simulink library "tqd"  (R2021b)
settings: Solver=VariableStepAuto  StartTime=0.0  StopTime=10.0  RelTol=1e-3
undefined symbols (not defined in the file or in its folder): ATQD_APSDecReq_X_kph, ATQD_APSDecReq_Y_mps2, ATQD_APSDecReqCMD_X_kph, ATQD_APSDecReqTs_X_pct, ATQD_APSDecTimeGain_X_Deg, ATQD_APSDecTimeGain_Y_s, ATQD_APSReqLowSpd_X_Deg, ATQD_AutoHoldReleaseBPS_X_Deg, ATQD_AWDLoadTrqnsGain_X_kg, ATQD_AWDLoadTrqnsGain_Y_pct, ATQD_BOSEnBPSPosn_X_kph, ATQD_BOSMap_X_rpm, ATQD_BOSMap_Y_pct, ATQD_CreepBaseTqD_X_kph, ATQD_CreepBaseTqD_Y_Deg, ATQD_CreepBaseTqR_X_kph, ATQD_CreepBaseTqR_Y_Deg, ATQD_CreepBPSDisPosn_X_Deg, ATQD_CreepBPSDisPosnR_X_Deg, ATQD_CreepBPSEnPosn_X_Deg, ATQD_CreepBPSEnPosnR_X_Deg, ATQD_CreepDeltaTq_X_kph, ATQD_CreepIterm_X_kph, ATQD_CreepIterm_Y_kph, ATQD_CreepItermMaxLimit_X_pct, ATQD_CreepPreloadTime_X_kph, ATQD_CreepPreloadTq_X_kph, ATQD_CreepPreloadTq_Y_s, ATQD_CreepProtTq_X_Deg, ATQD_CreepPterm_X_kph, ATQD_ECOTqMapD_X_rpm, ATQD_ECOTqMapD_Y_pct, ATQD_EOPDTqMapDCon_X_rpm, ATQD_EOPDTqMapDCon_Y_Deg, ATQD_EstInitVehWeight_X_c, ATQD_LHMRollGenMapD_X_rpm, ATQD_LHMRollGenMapD_Y_rpm, ATQD_LHMTqMapD_X_rpm, ATQD_LHMTqMapD_Y_pct, ATQD_NL1TqMapD_X_rpm, ATQD_NL1TqMapD_Y_pct, ATQD_NOPDTqMapDCon_X_rpm, ATQD_NOPDTqMapDCon_Y_Deg, ATQD_NRMRrEDUSpRat_X_rpm, ATQD_NRMRrEDUSpRat_Y_Nm, ATQD_OPDHoldDownRelDelay_X_Deg, ATQD_OPDHoldEnSpd_X_Deg, ATQD_OPDHoldRelDetTime_X_Deg, ATQD_OPDHoldReleaseTq_X_Deg, ATQD_OrigPedTqLowLim_X_Deg, ATQD_OrigPedTqLowLim_Y_pct, ATQD_PedalMapClimbUpLim_X_rpm, ATQD_PedalMapClimbUpLim_Y_Deg, ATQD_PreLoadTq_X_s, ATQD_RollGenMapEL1_X_rpm, ATQD_RollGenMapEL1_Y_rpm, ATQD_SL1TqMapD_X_rpm, ATQD_SL1TqMapD_Y_pct, ATQD_SlideRegenTqGain_X_Gps, ATQD_SlideRegenTqGain_Y_pct ... (+444)
libraries: hcu_lib x70, simulink x61, tqr x1
(part 1 of 14)
settings Model: Creator=13615  LastModifiedBy=FVT23010
settings SolverCC: AlgebraicLoopSolver=TrustRegion
settings DataIOCC: SaveFormat=Array  SignalLoggingSaveFormat=ModelDataLogs  ReturnWorkspaceOutputs=off
settings OptimizationCC: BlockReduction=off  BooleanDataType=off
settings DebuggingCC: SaveWithParameterizedLinksMsg=none  UnderspecifiedInitializationDetection=Classic  MergeDetectMultiDrivingBlocksExec=none  SignalResolutionControl=TryResolveAllWithWarning
settings HardwareCC: TargetUnknown=on
settings ModelReferenceCC: PropagateSignalLabelsOutOfModel=off
settings SFSimCC: SimUseLocalCustomCode=off
settings RTWCC: RTWUseLocalCustomCode=off
settings ConfigComp: CovMetricSettings=dw  CovSaveCumulativeToWorkspaceVar=on  CovSaveSingleToWorkspaceVar=on

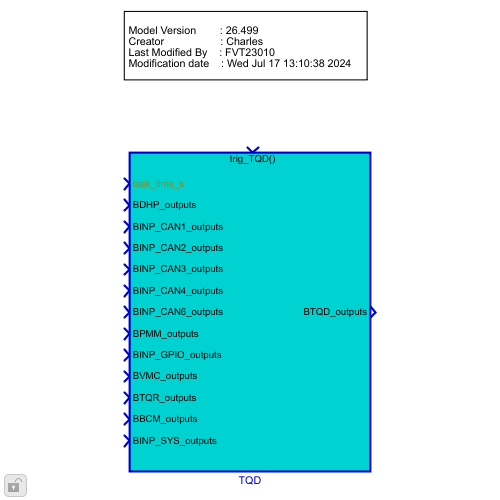
[thumbnail: Simulink's stored preview of the top-level diagram]
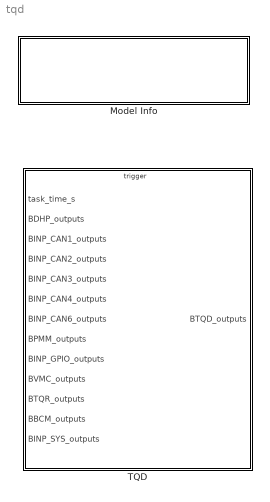
== system tqd ==
  Model Info : Subsystem  LoadFcn=slcm LoadBlock;  InitFcn=slcm('UpdateAllCMBlocksInThisModelInit')  mask(CMBlock){InitialSaveTempField=, InitialBlockCM=None, BlockCM=None, Frame=on, SaveTempField=, DisplayStringWithTags=|, MaskDisplayString=Model Version        : 26.504\nCreator                   : Charles\nLast Modified By    : FVT23010\nModification date    : Thu Jul 18 10:59:55 2024, HorizontalTextAlignment=Left, LeftAlignmentValue=0.02, SourceBlockDiagram=tqd, TagMaxNumber=20, CMTag1=, CMTag2=, CMTag3=, CMTag4=, CMTag5=, CMTag6=, CMTag7=, CMTag8=, CMTag9=, CMTag10=, CMTag11=, CMTag12=, CMTag13=, CMTag14=, CMTag15=, CMTag16=, CMTag17=, CMTag18=, CMTag19=, CMTag20=}
      mask DisplayStringWithTags=|
      | Model Version        : %<ModelVersion>
      | Creator                   : Charles
      | Last Modified By    : %<LastModifiedBy>
      | Modification date    : %<LastModificationDate>
      mask help: This block allows revision control information to be displayed within the model.
      settings: CopyFcn=slcm CopyBlock;  DeleteFcn=slcm Cancel;  PostSaveFcn=slcm('UpdateAllCMBlocksInThisModel')  NameChangeFcn=slcm Rename;  OpenFcn=slcm
      mask Display: text(str2num(LeftAlignmentValue), 0.5, MaskDisplayString, 'HorizontalAlignment', HorizontalTextAlignment)
  TQD : Subsystem
      settings: RTWSystemCode=Nonreusable function  RTWFcnNameOpts=Use subsystem name  RTWFileNameOpts=Use subsystem name

== system tqd/Model Info ==
  EmptySubsystem : Subsystem

== system tqd/TQD ==
  task_time_s : Inport
  BDHP_outputs : Inport  Port=2  OutDataTypeStr=Bus: BDHP_outputs
  BINP_CAN1_outputs : Inport  Port=3  OutDataTypeStr=Bus: BINP_CAN1_outputs
  BINP_CAN2_outputs : Inport  Port=4  OutDataTypeStr=Bus: BINP_CAN2_outputs
  BINP_CAN3_outputs : Inport  Port=5  OutDataTypeStr=Bus: BINP_CAN3_outputs
  BINP_CAN4_outputs : Inport  Port=6  OutDataTypeStr=Bus: BINP_CAN4_outputs
  BINP_CAN6_outputs : Inport  Port=7  OutDataTypeStr=Bus: BINP_CAN6_outputs
  BPMM_outputs : Inport  Port=8  OutDataTypeStr=Bus: BPMM_outputs
  BINP_GPIO_outputs : Inport  Port=9  OutDataTypeStr=Bus: BINP_GPIO_outputs
  BVMC_outputs : Inport  Port=10  OutDataTypeStr=Bus: BVMC_outputs
  BTQR_outputs : Inport  Port=11  OutDataTypeStr=Bus: BTQR_outputs  LockScale=on
  BBCM_outputs : Inport  Port=12  OutDataTypeStr=Bus: BBCM_outputs
  BINP_SYS_outputs : Inport  Port=13  OutDataTypeStr=Bus: BINP_SYS_outputs
  trig_TQD : TriggerPort  TriggerType=function-call  VariantControl=(inherit)
  Bus Creator2 : BusCreator  Inputs=87  OutDataTypeStr=Bus: BTQD_outputs  NonVirtualBus=on
  Bus Selector : BusSelector  OutputSignals=VINP_IVIPWModeReq_enum,VINP_IVICreepSWReq_flg,VINP_RollModeSWCmd_enum,VINP_IVIPwrLockSW_enum,VINP_IVIISAOffsetSpd_enum,VINP_Distanceunit_flg
  Bus Selector1 : BusSelector  OutputSignals=VDHP_ActAPSPosn_pct,VDHP_LowIdleAccPedal_flg
  Bus Selector10 : BusSelector  OutputSignals=VBCM_BrakeLamp_flg
  Bus Selector11 : BusSelector  OutputSignals=VINP_FlashRegenMode_enum
  Bus Selector12 : BusSelector  OutputSignals=VINP_ShifterHandleCmd_enum,VINP_FrEDURotateDirction_enum,VINP_RrEDURotateDirction_enum,VINP_FrTMSpd_rpm,VINP_RrTMSpd_rpm,VINP_HVBPwrAvailDchrg_kW,VINP_HVBPwrAvailChrg_kW,VINP_FrRegenAvailTq_Nm,VINP_RrRegenAvailTq_Nm,VINP_FrEDURealTMTq_Nm,VINP_RrEDURealTMTq_Nm,VINP_HVBattErr_flg,VINP_DCDCFaultSta_enum,VINP_FrMotorAvailTq_Nm,VINP_RrMotorAvailTq_Nm,VINP_MCUWarnF_enum,VINP_MCUWarnR_enum,VINP_ChrgPlugSta_enum,VINP_HVBCellVoltMax_mV,VINP_HVBCellVoltMin_mV,VINP_HVBSOH_pct,VINP_HVBattSOC_pct
  Bus Selector2 : BusSelector  OutputSignals=VINP_VehSpeed_kph,VINP_BrkSwSta_flg,VINP_BrkSwV_flg,VINP_BrkPedalPos_pct,VINP_BrkPedalPosSta_flg,VINP_FrPTCSActive_flg,VINP_RrPTCSActive_flg,VINP_FrntAxlTrqReqDrv_Nm,VINP_RearAxlTrqReqDrv_Nm,VINP_FrRBCActive_flg,VINP_RrRBCActive_flg,VINP_FrntAxlTrqReqBrk_Nm,VINP_RearAxlTrqReqBrk_Nm,VINP_CrashOutputSts_enum,VINP_LongAccel_Gps,VINP_EPBCarWashMode_flg,VINP_EPBErrSta_enum,VINP_EPBSta_enum,VINP_DOASta_flg,VINP_GRADE_Deg,VINP_HSAActive_flg,VINP_DriverSeatBeltCmd_flg,VINP_AVHActive_flg,VINP_PsngrSeatBeltCmd_flg,VINP_RDriverSeatBeltCmd_flg,VINP_RCenterSeatBeltCmd_flg,VINP_RPsngrSeatBeltCmd_flg,VINP_YawRate_degps,VINP_SASAngle_Deg,VINP_MCPressure_bar
  Bus Selector3 : BusSelector  OutputSignals=VINP_BrakeSWGPIO_flg,VINP_CrashSignalGPIO_flg,VINP_DrDoorSW_flg,VINP_SeatSW_flg,VINP_HoodSW_flg,VINP_TailgateSW_flg,VINP_PsDoorSW_flg,VINP_RRDoorSW_flg,VINP_RLDoorSW_flg
  Bus Selector5 : BusSelector  OutputSignals=VVMC_ADASForceIdle_flg,VVMC_ACCRequiredAccel_mps2,VVMC_ACCVehHoldReq_flg,VVMC_ADASActive_flg,VVMC_ADASWhlTqReq_Nm,VVMC_CruzActive_flg,VVMC_CruzWhlTqReq_Nm,VVMC_MSAActive_flg,VVMC_MSAWhlTqReq_Nm,VVMC_APSActive_flg,VVMC_APSSpeedCMD_kph,VVMC_APSShiftPosnReq_enum,VVMC_ACCPedalOvrd_flg,VVMC_LongAcc_Gps,VVMC_ActMaxSlideRate_pct,VVMC_EstSlope_Deg,VVMC_APSReq_enum,VVMC_RWDRDCActive_enum,VVMC_ActLRSlideRate_pct,VVMC_ActRRSlideRate_pct,VVMC_ActStESCYaw_Dps,VVMC_CCCtrlSta_enum,VVMC_MSACtrlSta_enum,VVMC_LVDAACCStatusInformation_flg,VVMC_ACCObjDist_m,VVMC_MeterIndSpeed_raw32,VVMC_RearTqRatio_rat,VVMC_ACCOvrdMemTq_Nm,VVMC_CalibratedGyroY_Dps,VVMC_CAASActive_flg
  Bus Selector6 : BusSelector  OutputSignals=VINP_SWCResUpSta_flg,VINP_SWCSetdownSta_flg,VINP_SWCACCSta_flg,VINP_SWCCANCELSta_flg,VINP_SWCRegenUp_flg,VINP_SWCRegenDown_flg
  Bus Selector7 : BusSelector  OutputSignals=VPMM_PowerSta_enum,VPMM_DrivetrainSelect_enum,VPMM_SysPowerMode_enum
  Bus Selector8 : BusSelector  OutputSignals=VTQR_ActualFEDUWhlTqReq_Nm,VTQR_ActualREDUWhlTqReq_Nm,VTQR_NoABSFEDUWhlTqReq_Nm,VTQR_NoABSREDUWhlTqReq_Nm
  Bus Selector9 : BusSelector  OutputSignals=VINP_ADASISASta_enum,VINP_ADASVehSpdLim_enum,VINP_ADASACCSta_enum
  Data Type Conversion : DataTypeConversion  OutDataTypeStr=uint8
  Data Type Conversion1 : DataTypeConversion  OutDataTypeStr=uint8
  Data Type Conversion2 : DataTypeConversion  OutDataTypeStr=boolean
  Data Type Conversion3 : DataTypeConversion  OutDataTypeStr=boolean
  Ground{,1..3} (4 alike) : Ground
  TorqueDemand : Subsystem
  BTQD_outputs : Outport  OutDataTypeStr=Bus: BTQD_outputs
  wires:
  Bus Selector2/19 -> TorqueDemand/25(VINP_DOASta_flg)  "<VINP_DOASta_flg>"
  Bus Selector2/18 -> TorqueDemand/24(VINP_EPBSta_enum)  "<VINP_EPBSta_enum>"
  Bus Selector2/17 -> TorqueDemand/23(VINP_EPBErrSta_enum)  "<VINP_EPBErrSta_enum>"
  Bus Selector2/16 -> TorqueDemand/22(VINP_EPBCarWashMode_flg)  "<VINP_EPBCarWashMode_flg>"
  Bus Selector2/15 -> TorqueDemand/21(VINP_LongAccel_Gps)  "<VINP_LongAccel_Gps>"
  BTQR_outputs/1 -> Bus Selector8/1
  Bus Selector2/14 -> TorqueDemand/20(VINP_CrashOutputSts_enum)  "<VINP_CrashOutputSts_enum>"
  TorqueDemand/8(VTQD_TqSourceFr_enum) -> Bus Creator2/8
  BDHP_outputs/1 -> Bus Selector1/1
  Bus Selector2/5 -> TorqueDemand/11(VINP_BrkPedalPosSta_flg)  "<VINP_BrkPedalPosSta_flg>"
  TorqueDemand/10(VTQD_FrEDUAvailBrkRgnTq_Nm) -> Bus Creator2/10
  TorqueDemand/9(VTQD_TqSourceRr_enum) -> Bus Creator2/9
  TorqueDemand/7(VTQD_AfterAvailableTqDemRr_Nm) -> Bus Creator2/7
  TorqueDemand/6(VTQD_AfterAvailableTqDemFr_Nm) -> Bus Creator2/6
  TorqueDemand/5(VTQD_DriverWhlTqDem_Nm) -> Bus Creator2/5
  Bus Selector/1 -> TorqueDemand/37(VINP_IVIPWModeReq_enum)  "<VINP_IVIPWModeReq_enum>"
  TorqueDemand/4(VTQD_PBWUnlockTO_flg) -> Bus Creator2/4
  TorqueDemand/3(VTQD_PBWLockTO_flg) -> Bus Creator2/3
  TorqueDemand/2(VTQD_ParkRequest_flg) -> Bus Creator2/2
  TorqueDemand/1(VTQD_GearActualPosn_enum) -> Bus Creator2/1
  BINP_CAN4_outputs/1 -> Bus Selector6/1  "BINP_CAN4_outputs"
  BINP_CAN2_outputs/1 -> Bus Selector/1  "BINP_CAN2_outputs"
  Bus Selector2/11 -> TorqueDemand/17(VINP_RrRBCActive_flg)  "<VINP_RrRBCActive_flg>"
  Bus Selector2/7 -> TorqueDemand/13(VINP_RrPTCSActive_flg)  "<VINP_RrPTCSActive_flg>"
  Bus Selector7/2 -> TorqueDemand/5(VPMM_DrivetrainSelect_enum)  "<VPMM_DrivetrainSelect_enum>"
  BINP_GPIO_outputs/1 -> Bus Selector3/1
  Bus Selector1/2 -> TorqueDemand/3(VDHP_LowIdleAccPedal_flg)  "<VDHP_LowIdleAccPedal_flg>"
  Bus Selector1/1 -> TorqueDemand/2(VDHP_ActAPSPosn_pct)  "<VDHP_ActAPSPosn_pct>"
  Bus Selector2/10 -> TorqueDemand/16(VINP_FrRBCActive_flg)  "<VINP_FrRBCActive_flg>"
  Bus Selector2/9 -> TorqueDemand/15(VINP_RearAxlTrqReqDrv_Nm)  "<VINP_RearAxlTrqReqDrv_Nm>"
  Bus Selector2/8 -> TorqueDemand/14(VINP_FrntAxlTrqReqDrv_Nm)  "<VINP_FrntAxlTrqReqDrv_Nm>"
  Bus Selector2/13 -> TorqueDemand/19(VINP_RearAxlTrqReqBrk_Nm)  "<VINP_RearAxlTrqReqBrk_Nm>"
  Bus Selector2/12 -> TorqueDemand/18(VINP_FrntAxlTrqReqBrk_Nm)  "<VINP_FrntAxlTrqReqBrk_Nm>"
  Bus Selector2/4 -> TorqueDemand/10(VINP_BrkPedalPos_pct)  "<VINP_BrkPedalPos_pct>"
  Bus Selector2/3 -> TorqueDemand/9(VINP_BrkSwV_flg)  "<VINP_BrkSwV_flg>"
  Bus Selector2/2 -> TorqueDemand/8(VINP_BrkSwSta_flg)  "<VINP_BrkSwSta_flg>"
  Bus Selector2/1 -> TorqueDemand/7(VINP_VehSpeed_kph)  "<VINP_VehSpeed_kph>"
  Bus Selector2/6 -> TorqueDemand/12(VINP_FrPTCSActive_flg)  "<VINP_FrPTCSActive_flg>"
  Bus Selector7/1 -> TorqueDemand/4(VPMM_PowerSta_enum)  "<VPMM_PowerSta_enum>"
  task_time_s/1 -> TorqueDemand/1(task_time_s)  "task_time_s"
  BINP_CAN3_outputs/1 -> Bus Selector12/1
  BINP_CAN1_outputs/1 -> Bus Selector2/1
  BPMM_outputs/1 -> Bus Selector7/1
  Bus Creator2/1 -> BTQD_outputs/1  "BTQD_outputs"
  Bus Selector2/20 -> TorqueDemand/26(VINP_GRADE_Deg)  "<VINP_GRADE_Deg>"
  Bus Selector2/21 -> TorqueDemand/27(VINP_HSAActive_flg)  "<VINP_HSAActive_flg>"
  Bus Selector/2 -> TorqueDemand/38(VINP_IVICreepSWReq_flg)  "<VINP_IVICreepSWReq_flg>"
  Bus Selector2/22 -> TorqueDemand/28(VINP_DriverSeatBeltCmd_flg)  "<VINP_DriverSeatBeltCmd_flg>"
  Bus Selector7/3 -> TorqueDemand/6(VPMM_SysPowerMode_enum)  "<VPMM_SysPowerMode_enum>"
  Bus Selector2/23 -> TorqueDemand/29(VINP_AVHActive_flg)  "<VINP_AVHActive_flg>"
  Bus Selector2/24 -> TorqueDemand/30(VINP_PsngrSeatBeltCmd_flg)  "<VINP_PsngrSeatBeltCmd_flg>"
  Bus Selector2/25 -> TorqueDemand/31(VINP_RDriverSeatBeltCmd_flg)  "<VINP_RDriverSeatBeltCmd_flg>"
  Bus Selector2/27 -> TorqueDemand/33(VINP_RPsngrSeatBeltCmd_flg)  "<VINP_RPsngrSeatBeltCmd_flg>"
  Bus Selector/3 -> TorqueDemand/39(VINP_RollModeSWCmd_enum)  "<VINP_RollModeSWCmd_enum>"
  Bus Selector2/26 -> TorqueDemand/32(VINP_RCenterSeatBeltCmd_flg)  "<VINP_RCenterSeatBeltCmd_flg>"
  Bus Selector6/1 -> TorqueDemand/65(VINP_SWCResUpSta_flg)  "<VINP_SWCResUpSta_flg>"
  Bus Selector/4 -> TorqueDemand/40(VINP_IVIPwrLockSW_enum)  "<VINP_IVIPwrLockSW_enum>"
  Ground2/1 -> Data Type Conversion/1
  Bus Selector2/28 -> TorqueDemand/34(VINP_YawRate_degps)  "<VINP_YawRate_degps>"
  Bus Selector2/29 -> TorqueDemand/35(VINP_SASAngle_Deg)  "<VINP_SASAngle_Deg>"
  Bus Selector2/30 -> TorqueDemand/36(VINP_MCPressure_bar)  "<VINP_MCPressure_bar>"
  TorqueDemand/11(VTQD_RrEDUAvailBrkRgnTq_Nm) -> Bus Creator2/11
  TorqueDemand/12(VTQD_TqTargetShaftSpd_rpm) -> Bus Creator2/12
  TorqueDemand/13(VTQD_LimpHomeAct_flg) -> Bus Creator2/13
  TorqueDemand/14(VTQD_RollRegenEnable_flg) -> Bus Creator2/14
  TorqueDemand/15(VTQD_EVDriveMode_enum) -> Bus Creator2/15
  TorqueDemand/16(VTQD_EVDriveModeValid_flg) -> Bus Creator2/16
  TorqueDemand/17(VTQD_ShiftGearPosn_enum) -> Bus Creator2/17
  TorqueDemand/18(VTQD_PButtonSta_enum) -> Bus Creator2/18
  TorqueDemand/19(VTQD_FrActvDmpDisabReq_flg) -> Bus Creator2/19
  TorqueDemand/20(VTQD_RrActvDmpDisabReq_flg) -> Bus Creator2/20
  TorqueDemand/21(VTQD_FrRgnDecrSta_flg) -> Bus Creator2/21
  TorqueDemand/22(VTQD_RrRgnDecrSta_flg) -> Bus Creator2/22
  TorqueDemand/23(VTQD_DriverWhlTqDemFr_Nm) -> Bus Creator2/23
  TorqueDemand/24(VTQD_DriverWhlTqDemRr_Nm) -> Bus Creator2/24
  TorqueDemand/25(VTQD_FrEDUActTq_Nm) -> Bus Creator2/25
  TorqueDemand/26(VTQD_RrEDUActTq_Nm) -> Bus Creator2/26
  TorqueDemand/27(VTQD_FrEDURolRgnTq_Nm) -> Bus Creator2/27
  TorqueDemand/28(VTQD_RrEDURolRgnTq_Nm) -> Bus Creator2/28
  TorqueDemand/29(VTQD_FrEDUSpd_rpm) -> Bus Creator2/29
  TorqueDemand/30(VTQD_RrEDUSpd_rpm) -> Bus Creator2/30
  TorqueDemand/31(VTQD_FrEDUSpdValid_flg) -> Bus Creator2/31
  TorqueDemand/32(VTQD_FrEDUAvailBrkRgnTqV_flg) -> Bus Creator2/32
  TorqueDemand/33(VTQD_RrEDUSpdValid_flg) -> Bus Creator2/33
  TorqueDemand/34(VTQD_RrEDUAvailBrkRgnTqV_flg) -> Bus Creator2/34
  TorqueDemand/35(VTQD_RgnAbnorSta_flg) -> Bus Creator2/35
  TorqueDemand/36(VTQD_PTCSPermSta_flg) -> Bus Creator2/36
  TorqueDemand/37(VTQD_FrRgnPermSta_flg) -> Bus Creator2/37
  TorqueDemand/38(VTQD_RrRgnPermSta_flg) -> Bus Creator2/38
  TorqueDemand/39(VTQD_ExternalTqAllow_flg) -> Bus Creator2/39
  TorqueDemand/40(VTQD_FrIdcMin_A) -> Bus Creator2/40
  TorqueDemand/41(VTQD_FrIdcMax_A) -> Bus Creator2/41
  TorqueDemand/42(VTQD_FrUdcMin_V) -> Bus Creator2/42
  TorqueDemand/43(VTQD_FrUdcMax_V) -> Bus Creator2/43
  TorqueDemand/44(VTQD_RrIdcMin_A) -> Bus Creator2/44
  TorqueDemand/45(VTQD_RrIdcMax_A) -> Bus Creator2/45
  TorqueDemand/46(VTQD_RrUdcMin_V) -> Bus Creator2/46
  TorqueDemand/47(VTQD_RrUdcMax_V) -> Bus Creator2/47
  TorqueDemand/48(VTQD_CoordWhlTqDemFr_Nm) -> Bus Creator2/48
  TorqueDemand/49(VTQD_CoordWhlTqDemRr_Nm) -> Bus Creator2/49
  TorqueDemand/50(VTQD_CreepEnable_flg) -> Bus Creator2/50
  TorqueDemand/51(VTQD_CrashDetd_flg) -> Bus Creator2/51
  TorqueDemand/52(VTQD_DiagHCrash_flg) -> Bus Creator2/52
  TorqueDemand/53(VTQD_ReBrakeLPReq_flg) -> Bus Creator2/53
  TorqueDemand/54(VTQD_LoSpdBrkCtrl_flg) -> Bus Creator2/54
  TorqueDemand/55(VTQD_LowIdleAccPedal_flg) -> Bus Creator2/55
  TorqueDemand/56(VTQD_APSStaSys_enum) -> Bus Creator2/56
  TorqueDemand/57(VTQD_APSReq_enum) -> Bus Creator2/57
  TorqueDemand/58(VTQD_APSDecReqA_flg) -> Bus Creator2/58
  TorqueDemand/59(VTQD_APSDecReq_mps2) -> Bus Creator2/59
  TorqueDemand/60(VTQD_ExtShftAllow_flg) -> Bus Creator2/60
  TorqueDemand/61(VTQD_EstVehWeightResult_kg) -> Bus Creator2/61
  TorqueDemand/62(VTQD_BOSEnable_flg) -> Bus Creator2/62
  TorqueDemand/63(VTQD_CreepON_flg) -> Bus Creator2/63
  TorqueDemand/64(VTQD_PreLoadHold_flg) -> Bus Creator2/64
  TorqueDemand/65(VTQD_PreLoadPreEn_flg) -> Bus Creator2/65
  TorqueDemand/66(VTQD_CreepPrLoadEnable_flg) -> Bus Creator2/66
  TorqueDemand/67(VTQD_RDCActive_enum) -> Bus Creator2/67
  TorqueDemand/68(VTQD_EquivAccPedalSWSta_flg) -> Bus Creator2/68
  TorqueDemand/69(VTQD_DriveProtEn_flg) -> Bus Creator2/69
  TorqueDemand/70(VTQD_ActParkRequest_flg) -> Bus Creator2/70
  TorqueDemand/71(VTQD_RegenTqLimitEn_flg) -> Bus Creator2/71
  TorqueDemand/72(VTQD_PedAccTqEn_flg) -> Bus Creator2/72
  TorqueDemand/73(VTQD_IVIPwrLockSta_enum) -> Bus Creator2/73
  TorqueDemand/74(VTQD_ExtDoorAllow_flg) -> Bus Creator2/74
  TorqueDemand/75(VTQD_WhlTqCapGenFr_Nm) -> Bus Creator2/75
  TorqueDemand/76(VTQD_WhlTqCapGenRr_Nm) -> Bus Creator2/76
  TorqueDemand/77(VTQD_OPDHoldLamp_flg) -> Bus Creator2/77
  TorqueDemand/78(VTQD_RegenMode_enum) -> Bus Creator2/78
  BINP_CAN6_outputs/1 -> Bus Selector9/1
  Bus Selector/5 -> TorqueDemand/41(VINP_IVIISAOffsetSpd_enum)  "<VINP_IVIISAOffsetSpd_enum>"
  BBCM_outputs/1 -> Bus Selector10/1
  Bus Selector6/2 -> TorqueDemand/66(VINP_SWCSetdownSta_flg)  "<VINP_SWCSetdownSta_flg>"
  Bus Selector6/3 -> TorqueDemand/67(VINP_SWCACCSta_flg)  "<VINP_SWCACCSta_flg>"
  Bus Selector6/4 -> TorqueDemand/68(VINP_SWCCANCELSta_flg)  "<VINP_SWCCANCELSta_flg>"
  Bus Selector6/5 -> TorqueDemand/69(VINP_SWCRegenUp_flg)  "<VINP_SWCRegenUp_flg>"
  Bus Selector6/6 -> TorqueDemand/70(VINP_SWCRegenDown_flg)  "<VINP_SWCRegenDown_flg>"
  TorqueDemand/79(VTQD_SaveRegenMode_enum) -> Bus Creator2/79
  TorqueDemand/80(VTQD_FDCVCURegenMode_enum) -> Bus Creator2/80
  TorqueDemand/81(VTQD_SpdCtrlMode_enum) -> Bus Creator2/81
  TorqueDemand/82(VTQD_SpdCtrlSta_flg) -> Bus Creator2/82
  TorqueDemand/83(VTQD_SetSpd_kph) -> Bus Creator2/83
  BINP_SYS_outputs/1 -> Bus Selector11/1
  TorqueDemand/84(VTQD_SWCCancelSta_flg) -> Bus Creator2/84
  TorqueDemand/85(VTQD_SWCSetdownSta_flg) -> Bus Creator2/85
  TorqueDemand/86(VTQD_SWCResUpSta_flg) -> Bus Creator2/86
  Bus Selector/6 -> TorqueDemand/42(VINP_Distanceunit_flg)  "<VINP_Distanceunit_flg>"
  Bus Selector12/1 -> TorqueDemand/43(VINP_ShifterHandleCmd_enum)  "<VINP_ShifterHandleCmd_enum>"
  Bus Selector12/2 -> TorqueDemand/44(VINP_FrEDURotateDirction_enum)  "<VINP_FrEDURotateDirction_enum>"
  Bus Selector12/3 -> TorqueDemand/45(VINP_RrEDURotateDirction_enum)  "<VINP_RrEDURotateDirction_enum>"
  Bus Selector12/4 -> TorqueDemand/46(VINP_FrTMSpd_RPM)  "<VINP_FrTMSpd_rpm>"
  Bus Selector12/5 -> TorqueDemand/47(VINP_RrTMSpd_RPM)  "<VINP_RrTMSpd_rpm>"
  Bus Selector12/6 -> TorqueDemand/48(VINP_HVBPwrAvailDchrg_kw)  "<VINP_HVBPwrAvailDchrg_kW>"
  Bus Selector12/7 -> TorqueDemand/49(VINP_HVBPwrAvailChrg_kw)  "<VINP_HVBPwrAvailChrg_kW>"
  Bus Selector12/8 -> TorqueDemand/50(VINP_FrRegenAvailTq_Nm)  "<VINP_FrRegenAvailTq_Nm>"
  Bus Selector12/9 -> TorqueDemand/51(VINP_RrRegenAvailTq_Nm)  "<VINP_RrRegenAvailTq_Nm>"
  Bus Selector12/10 -> TorqueDemand/52(VINP_FrEDURealTMTq_Nm)  "<VINP_FrEDURealTMTq_Nm>"
  Bus Selector12/11 -> TorqueDemand/53(VINP_RrEDURealTMTq_Nm)  "<VINP_RrEDURealTMTq_Nm>"
  Bus Selector12/12 -> TorqueDemand/54(VINP_HVBattErr_flg)  "<VINP_HVBattErr_flg>"
  Bus Selector12/13 -> TorqueDemand/55(VINP_DCDCFaultSta_enum)  "<VINP_DCDCFaultSta_enum>"
  Bus Selector12/14 -> TorqueDemand/56(VINP_FrMotorAvailTq_Nm)  "<VINP_FrMotorAvailTq_Nm>"
  Bus Selector12/15 -> TorqueDemand/57(VINP_RrMotorAvailTq_Nm)  "<VINP_RrMotorAvailTq_Nm>"
  Bus Selector12/16 -> TorqueDemand/58(VINP_MCUWarnF_enum)  "<VINP_MCUWarnF_enum>"
  Bus Selector12/17 -> TorqueDemand/59(VINP_MCUWarnR_enum)  "<VINP_MCUWarnR_enum>"
  Bus Selector12/18 -> TorqueDemand/60(VINP_ChrgPlugSta_enum)  "<VINP_ChrgPlugSta_enum>"
  Bus Selector12/19 -> TorqueDemand/61(VINP_HVBCellVoltMax_mV)  "<VINP_HVBCellVoltMax_mV>"
  Bus Selector12/20 -> TorqueDemand/62(VINP_HVBCellVoltMin_mV)  "<VINP_HVBCellVoltMin_mV>"
  Bus Selector12/21 -> TorqueDemand/63(VINP_HVBSOH_pct)  "<VINP_HVBSOH_pct>"
  Bus Selector12/22 -> TorqueDemand/64(VINP_HVBattSOC_pct)  "<VINP_HVBattSOC_pct>"
  TorqueDemand/87(VTQD_CreepBaseTqD_Nm) -> Bus Creator2/87
  Bus Selector5/1 -> TorqueDemand/72(VINP_ADASForceIdle_flg)  "<VVMC_ADASForceIdle_flg>"
  Bus Selector5/2 -> TorqueDemand/73(VINP_ACCRequiredAccel_mps2)  "<VVMC_ACCRequiredAccel_mps2>"
  Bus Selector5/3 -> TorqueDemand/74(VINP_ACCVehHoldReq_flg)  "<VVMC_ACCVehHoldReq_flg>"
  Bus Selector5/4 -> TorqueDemand/75(VVMC_ADASActive_flg)  "<VVMC_ADASActive_flg>"
  Bus Selector5/5 -> TorqueDemand/76(VVMC_ADASWhlTqReq_Nm)  "<VVMC_ADASWhlTqReq_Nm>"
  Bus Selector5/6 -> TorqueDemand/77(VVMC_CruzActive_flg)  "<VVMC_CruzActive_flg>"
  Bus Selector5/7 -> TorqueDemand/78(VVMC_CruzWhlTqReq_Nm)  "<VVMC_CruzWhlTqReq_Nm>"
  Bus Selector5/8 -> TorqueDemand/79(VVMC_MSAActive_flg)  "<VVMC_MSAActive_flg>"
  Bus Selector5/9 -> TorqueDemand/80(VVMC_MSAWhlTqReq_Nm)  "<VVMC_MSAWhlTqReq_Nm>"
  Bus Selector5/10 -> TorqueDemand/81(VVMC_APSActive_flg)  "<VVMC_APSActive_flg>"
  Bus Selector5/11 -> TorqueDemand/82(VVMC_APSSpeedCMD_kph)  "<VVMC_APSSpeedCMD_kph>"
  Bus Selector5/12 -> TorqueDemand/83(VVMC_APSShiftPosnReq_enum)  "<VVMC_APSShiftPosnReq_enum>"
  Bus Selector5/13 -> TorqueDemand/84(VVMC_ACCPedalOvrd_flg)  "<VVMC_ACCPedalOvrd_flg>"
  Bus Selector5/14 -> TorqueDemand/85(VVMC_LongAcc_Gps)  "<VVMC_LongAcc_Gps>"
  Bus Selector5/15 -> TorqueDemand/86(VVMC_ActMaxSlideRate_pct)  "<VVMC_ActMaxSlideRate_pct>"
  Bus Selector5/16 -> TorqueDemand/87(VVMC_EstSlope_Deg)  "<VVMC_EstSlope_Deg>"
  Bus Selector5/17 -> TorqueDemand/88(VVMC_APSReq_enum)  "<VVMC_APSReq_enum>"
  Bus Selector5/18 -> TorqueDemand/89(VVMC_RWDRDCActive_enum)  "<VVMC_RWDRDCActive_enum>"
  Bus Selector5/19 -> TorqueDemand/90(VVMC_ActLRSlideRate_pct)  "<VVMC_ActLRSlideRate_pct>"
  Bus Selector5/20 -> TorqueDemand/91(VVMC_ActRRSlideRate_pct)  "<VVMC_ActRRSlideRate_pct>"
  Bus Selector5/21 -> TorqueDemand/92(VVMC_ActStESCYaw_degps)  "<VVMC_ActStESCYaw_Dps>"
  Bus Selector5/22 -> TorqueDemand/93(VVMC_CCCtrlSta_enum)  "<VVMC_CCCtrlSta_enum>"
  Bus Selector5/23 -> TorqueDemand/94(VVMC_MSACtrlSta_enum)  "<VVMC_MSACtrlSta_enum>"
  Bus Selector5/24 -> TorqueDemand/95(VVMC_LVDAACCStatusInformation_flg)  "<VVMC_LVDAACCStatusInformation_flg>"
  Bus Selector5/25 -> TorqueDemand/96(VVMC_ACCObjDist_m)  "<VVMC_ACCObjDist_m>"
  Bus Selector5/26 -> TorqueDemand/97(VVMC_MeterIndSpeed_raw32)  "<VVMC_MeterIndSpeed_raw32>"
  Bus Selector5/27 -> TorqueDemand/98(VVMC_RearTqRatio_rat)  "<VVMC_RearTqRatio_rat>"
  Bus Selector5/28 -> TorqueDemand/99(VVMC_ACCOvrdMemTq_Nm)  "<VVMC_ACCOvrdMemTq_Nm>"
  Bus Selector5/29 -> TorqueDemand/100(VVMC_CalibratedGyroY_Dps)  "<VVMC_CalibratedGyroY_Dps>"
  Bus Selector5/30 -> TorqueDemand/101(VVMC_CAASActive_flg)  "<VVMC_CAASActive_flg>"
  BVMC_outputs/1 -> Bus Selector5/1
  Bus Selector3/1 -> TorqueDemand/102(VINP_BrakeSWGPIO_flg)  "<VINP_BrakeSWGPIO_flg>"
  Bus Selector3/2 -> TorqueDemand/103(VINP_CrashSignalGPIO_flg)  "<VINP_CrashSignalGPIO_flg>"
  Bus Selector3/3 -> TorqueDemand/104(VINP_DrDoorSW_flg)  "<VINP_DrDoorSW_flg>"
  Bus Selector3/4 -> TorqueDemand/105(VINP_SeatSW_flg)  "<VINP_SeatSW_flg>"
  Bus Selector3/5 -> TorqueDemand/106(VINP_HoodSW_flg)  "<VINP_HoodSW_flg>"
  Bus Selector3/6 -> TorqueDemand/107(VINP_TailgateSW_flg)  "<VINP_TailgateSW_flg>"
  Bus Selector3/7 -> TorqueDemand/108(VINP_PsDoorSW_flg)  "<VINP_PsDoorSW_flg>"
  Bus Selector3/8 -> TorqueDemand/109(VINP_RRDoorSW_flg)  "<VINP_RRDoorSW_flg>"
  Bus Selector3/9 -> TorqueDemand/110(VINP_RLDoorSW_flg)  "<VINP_RLDoorSW_flg>"
  Bus Selector8/1 -> TorqueDemand/111(VTQR_ActualFEDUWhlTqReq_Nm)  "<VTQR_ActualFEDUWhlTqReq_Nm>"
  Bus Selector8/2 -> TorqueDemand/112(VTQR_ActualREDUWhlTqReq_Nm)  "<VTQR_ActualREDUWhlTqReq_Nm>"
  Bus Selector8/3 -> TorqueDemand/113(VTQR_NoABSFEDUWhlTqReq_Nm)  "<VTQR_NoABSFEDUWhlTqReq_Nm>"
  Bus Selector8/4 -> TorqueDemand/114(VTQR_NoABSREDUWhlTqReq_Nm)  "<VTQR_NoABSREDUWhlTqReq_Nm>"
  Ground/1 -> Data Type Conversion2/1
  Ground3/1 -> Data Type Conversion3/1
  Ground1/1 -> Data Type Conversion1/1
  Data Type Conversion/1 -> TorqueDemand/71(VINP_SCPSystemMode_enum)
  Data Type Conversion1/1 -> TorqueDemand/115(VINP_PBWMotorPos_enum)
  Data Type Conversion2/1 -> TorqueDemand/116(VDDM_LimpHomeAct_flg)
  Data Type Conversion3/1 -> TorqueDemand/117(VINP_CreepSW_flg)
  Bus Selector10/1 -> TorqueDemand/118(VBCM_BrakeLamp_flg)  "<VBCM_BrakeLamp_flg>"
  Bus Selector9/1 -> TorqueDemand/119(VINP_ADASISASta_enum)  "<VINP_ADASISASta_enum>"
  Bus Selector9/2 -> TorqueDemand/120(VINP_ADASVehSpdLim_kph)  "<VINP_ADASVehSpdLim_enum>"
  Bus Selector9/3 -> TorqueDemand/121(VINP_ADASACCSta_enum)  "<VINP_ADASACCSta_enum>"
  Bus Selector11/1 -> TorqueDemand/122(VINP_FlashRegenMode_enum)  "<VINP_FlashRegenMode_enum>"

== system tqd/Model Info/EmptySubsystem ==
